simulink model "sim_P_LOS"  (R2017a)
settings: Solver=FixedStepAuto  StartTime=0.0  StopTime=inf  FixedStep=0.01  RelTol=1e-3
values from neighbouring files (symbols this model uses):
  trial_params = sim_params(i)    [exec_sim_main.m]
libraries: simulink x4, emily x1
settings Model: Creator=mitchallain  LastModifiedBy=mitchallain
settings DataIOCC: SaveOutput=off  SaveTime=off

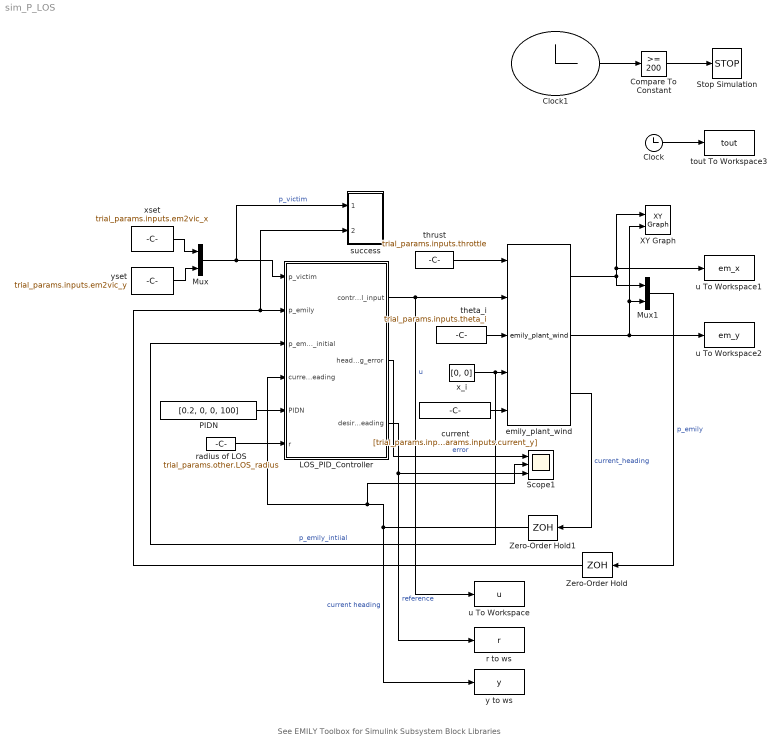
== system sim_P_LOS ==
  note: See EMILY Toolbox for Simulink Subsystem Block Libraries
  Clock : Clock
  Clock1 : Clock
  Compare To Constant : simulink/Logic and Bit Operations/Compare To Constant  relop=>=  const=200  OutDataTypeStr=boolean
  LOS_PID_Controller : Subsystem  AncestorBlock=emily/LOS_PID_Controller
      settings: AttributesFormatString=%<LinkStatus>
  Mux : Mux  Inputs=2
  Mux1 : Mux  Inputs=2
  PIDN : Constant  Value=[0.2, 0, 0, 100]
  Scope1 : Scope  NumInputPorts=3
  Stop Simulation : Stop
  XY Graph : simulink/Sinks/XY Graph  xmin=-50  xmax=50  ymin=-50  ymax=50  st=-1
  Zero-Order Hold : ZeroOrderHold  SampleTime=0.2
  Zero-Order Hold1 : ZeroOrderHold  SampleTime=0.2
  current : Constant  Value=[trial_params.inputs.current_x, trial_params.inputs.current_y]
  emily_plant_wind : emily/emily_plant_wind
      settings: SourceProductName=EMILY Toolbox
  r to ws : ToWorkspace  VariableName=r  SampleTime=0.2
  radius of LOS : Constant  Value=trial_params.other.LOS_radius
  success : Subsystem  AncestorBlock=emily/success
  theta_i : Constant  Value=trial_params.inputs.theta_i
  thrust : Constant  Value=trial_params.inputs.throttle
  tout To Workspace3 : ToWorkspace  VariableName=tout  SampleTime=0.2
  u To Workspace : ToWorkspace  VariableName=u  SampleTime=0.2
  u To Workspace1 : ToWorkspace  VariableName=em_x  SampleTime=0.2
  u To Workspace2 : ToWorkspace  VariableName=em_y  SampleTime=0.2
  x_i : Constant  Value=[0, 0]
  xset : Constant  Value=trial_params.inputs.em2vic_x
  y to ws : ToWorkspace  VariableName=y  SampleTime=0.2
  yset : Constant  Value=trial_params.inputs.em2vic_y
  wires:
  emily_plant_wind/1 -> XY Graph/1, u To Workspace1/1, Mux1/1
  Mux1/1 -> Zero-Order Hold/1  "p_emily"
  thrust/1 -> emily_plant_wind/1
  Mux/1 -> LOS_PID_Controller/1(p_victim), success/1(p_victim)  "p_victim"
  theta_i/1 -> emily_plant_wind/3
  emily_plant_wind/3 -> Zero-Order Hold1/1  "current_heading"
  xset/1 -> Mux/1
  yset/1 -> Mux/2
  emily_plant_wind/2 -> XY Graph/2, Mux1/2, u To Workspace2/1
  LOS_PID_Controller/2(heading_error) -> Scope1/1  "error"
  LOS_PID_Controller/1(control_input) -> emily_plant_wind/2, u To Workspace/1  "u"
  LOS_PID_Controller/3(desired_heading) -> Scope1/3, r to ws/1  "reference"
  x_i/1 -> LOS_PID_Controller/3(p_emily_initial), emily_plant_wind/4  "p_emily_intiial"
  Zero-Order Hold/1 -> LOS_PID_Controller/2(p_emily), success/2(p_emily)
  Zero-Order Hold1/1 -> Scope1/2, LOS_PID_Controller/4(current_heading), y to ws/1  "current heading"
  current/1 -> emily_plant_wind/5
  Clock/1 -> tout To Workspace3/1
  radius of LOS/1 -> LOS_PID_Controller/6(r)
  PIDN/1 -> LOS_PID_Controller/5(PIDN)
  Clock1/1 -> Compare To Constant/1
  Compare To Constant/1 -> Stop Simulation/1

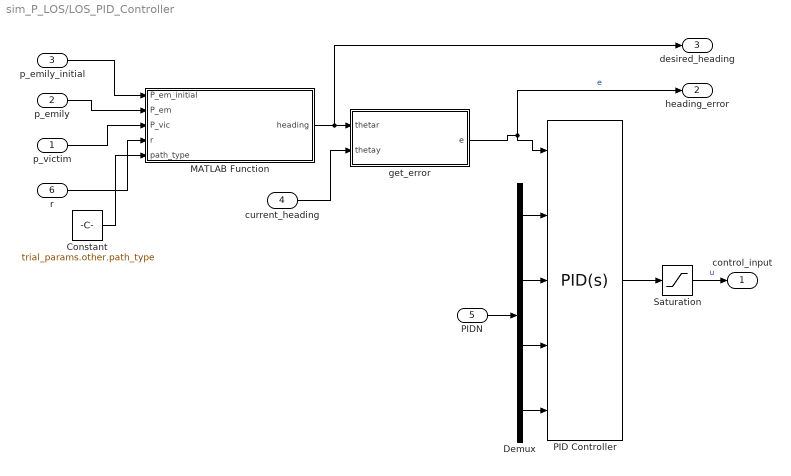
== system sim_P_LOS/LOS_PID_Controller ==
  p_victim : Inport
  p_emily : Inport  Port=2
  p_emily_initial : Inport  Port=3
  current_heading : Inport  Port=4
  PIDN : Inport  Port=5
  r : Inport  Port=6
  Constant : Constant  Value=trial_params.other.path_type  SampleTime=-1
  Demux : Demux
  MATLAB Function : MATLAB Function  TreatAsAtomicUnit=on
  PID Controller : simulink/Continuous/PID Controller  Controller=PID  TimeDomain=Continuous-time  SampleTime=-1  IntegratorMethod=Forward Euler  FilterMethod=Forward Euler  Form=Parallel  UseFilter=on  ControllerParametersSource=external  P=0.01  I=0.0001  D=1  N=100  InitialConditionSource=internal  InitialConditionForIntegrator=0  InitialConditionForFilter=0  ExternalReset=none  LimitOutput=off  UpperSaturationLimit=pi/4  LowerSaturationLimit=-pi/4  LinearizeAsGain=on  AntiWindupMode=clamping  Kb=1  TrackingMode=off  Kt=1  PParamMin=[]  PParamMax=[]  IParamMin=[]  IParamMax=[]  DParamMin=[]  DParamMax=[]  NParamMin=[]  NParamMax=[]  KbParamMin=[]  KbParamMax=[]  KtParamMin=[]  KtParamMax=[]  POutMin=[]  POutMax=[]  IOutMin=[]  IOutMax=[]  DOutMin=[]  DOutMax=[]  NOutMin=[]  NOutMax=[]  KbOutMin=[]  KbOutMax=[]  KtOutMin=[]  KtOutMax=[]  IntegratorOutMin=[]  IntegratorOutMax=[]  FilterOutMin=[]  FilterOutMax=[]  SumOutMin=[]  SumOutMax=[]  SumI1OutMin=[]  SumI1OutMax=[]  SumI2OutMin=[]  SumI2OutMax=[]  SumI3OutMin=[]  SumI3OutMax=[]  SumDOutMin=[]  SumDOutMax=[]  SaturationOutMin=[]  SaturationOutMax=[]  IntegratorContinuousStateAttributes=''  IntegratorStateMustResolveToSignalObject=off  IntegratorRTWStateStorageClass=Auto  FilterContinuousStateAttributes=''  FilterStateMustResolveToSignalObject=off  FilterRTWStateStorageClass=Auto  DifferentiatorICPrevScaledInput=0  DifferentiatorOutMin=[]  DifferentiatorOutMax=[]  InitialConditionSetting=State (most efficient)
  Saturation : Saturate  UpperLimit=pi/4  LowerLimit=-pi/4
  get_error : MATLAB Function  TreatAsAtomicUnit=on
  control_input : Outport
  heading_error : Outport  Port=2
  desired_heading : Outport  Port=3
  wires:
  r/1 -> MATLAB Function/4(r)
  p_emily_initial/1 -> MATLAB Function/1(P_em_initial)
  p_emily/1 -> MATLAB Function/2(P_em)
  p_victim/1 -> MATLAB Function/3(P_vic)
  Demux/4 -> PID Controller/5
  Demux/3 -> PID Controller/4
  Demux/2 -> PID Controller/3
  Demux/1 -> PID Controller/2
  PIDN/1 -> Demux/1
  current_heading/1 -> get_error/2(thetay)
  get_error/1(e) -> PID Controller/1, heading_error/1  "e"
  PID Controller/1 -> Saturation/1
  Saturation/1 -> control_input/1  "u"
  Constant/1 -> MATLAB Function/5(path_type)
  MATLAB Function/1(heading) -> get_error/1(thetar), desired_heading/1

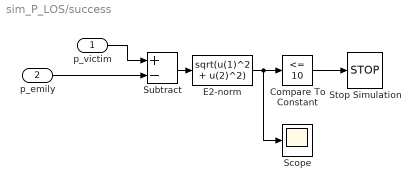
== system sim_P_LOS/success ==
  p_victim : Inport
  p_emily : Inport  Port=2
  Compare To Constant : simulink/Logic and Bit Operations/Compare To Constant  relop=<=  const=10  OutDataTypeStr=boolean
  E2-norm : Fcn  Expr=sqrt(u(1)^2 + u(2)^2)
  Scope : Scope
  Stop Simulation : Stop
  Subtract : Sum  Inputs=+-
  wires:
  Subtract/1 -> E2-norm/1
  E2-norm/1 -> Compare To Constant/1, Scope/1
  p_victim/1 -> Subtract/1
  Compare To Constant/1 -> Stop Simulation/1
  p_emily/1 -> Subtract/2

== matlab function sim_P_LOS/LOS_PID_Controller/get_error ==
  data: thetar input; e output; thetay input
function e  = get_error(thetar, thetay)
%UNTITLED Summary of this function goes here
%   FIX THIS MITCH
e = thetar - thetay;
e = mod((e + pi), 2*pi) - pi;
end

== matlab function sim_P_LOS/LOS_PID_Controller/MATLAB Function ==
  data: P_em_initial input; heading output; P_em input; P_vic input; r input; path_type input
function heading  = straightpathLOS(P_em_initial, P_em, P_vic, r, path_type)
% This function computes the heading angle according to LOS geometric law
%   Assumes straight line path from initial location to victim
%   If two intersections are produced, the intersection with a higher
%   dispacement parameter (s) is chosen (i.e., farther along path)

% Args:
%   P_em_initial (2-vector): initial (x, y) location of EMILY
%   P_em (2-vector): current (x, y) location of EMILY
%   P_vic (2-vector): victim (x, y) location
%   r (float): radius for LOS control

% Returns:
%   heading: heading angle for EMILY in global frame

% Compute vector from initial EMILY to victim in global frame
P_eiv = P_vic - P_em_initial;

% Compute desired path length and angle
d = norm(P_eiv);
path_angle = atan2(P_eiv(2), P_eiv(1));

% Compute vector from current EMILY to victim
P_ev = P_vic - P_em;

% Bearing is used to seed the fminsearch
bearing = atan2(P_ev(2), P_ev(1));

% Parameterized circle about emily
xLOS = @(phi) P_em(1) + r*cos(phi);
yLOS = @(phi) P_em(2) + r*sin(phi);

switch path_type
    case 1
        x = [P_em_initial(1) P_vic(1)/3  P_vic(1)*2/3  P_vic(1)]; %spline intersection pts
        y = [P_em_initial(2) P_vic(2)*2/3  P_vic(2)*2/3  P_vic(2)];
        pp = spline(x,y);
        path = @(s) ppval(pp,s);
        xy = @(param) (path(param(1)) - xLOS(param(2)))^2 + (path(param(1)) - yLOS(param(2)))^2;
        temp = fminsearch(@(param) xy(param), [P_em(1)+20*cos(bearing), bearing]);
        s_i = temp(1);
        phi_i = temp(2);
        P_es = [s_i - P_em(1); path(s_i) - P_em(2)];
        
    case 2
        x = [P_em_initial(1) P_vic(1)/3 P_vic(1)*2/3 P_vic(1)]; %spline intersection pts
        y = [P_em_initial(2) P_em_initial(2)*4/3 P_vic(2)/3  P_vic(2)];
        pp = spline(x,y);
        path = @(s) ppval(pp,s);
        xy = @(param) (path(param(1)) - xLOS(param(2)))^2 + (path(param(1)) - yLOS(param(2)))^2;
        temp = fminsearch(@(param) xy(param), [P_em(1)+20*cos(bearing), bearing]);
        s_i = temp(1);
        phi_i = temp(2);
        P_es = [s_i - P_em(1); path(s_i) - P_em(2)];
        
    case 3
        x = [P_em_initial(1) P_vic(1)/3 P_vic(1)*2/3 P_vic(1)]; %spline intersection pts
        y = [P_em_initial(2) P_vic(2)*2/3 P_em_initial(2)*4/3  P_vic(2)];
        pp = spline(x,y);
        path = @(s) ppval(pp,s);
        xy = @(param) (path(param(1)) - xLOS(param(2)))^2 + (path(param(1)) - yLOS(param(2)))^2;
        temp = fminsearch(@(param) xy(param), [P_em(1)+20*cos(bearing), bearing]);
        s_i = temp(1);
        phi_i = temp(2);
        P_es = [s_i - P_em(1); path(s_i) - P_em(2)];

    otherwise %'straight'
        xpath = @(s) P_em_initial(1) + s*cos(path_angle);
        ypath = @(s) P_em_initial(2) + s*sin(path_angle);
        xy = @(param) (xpath(param(1)) - xLOS(param(2)))^2 + (ypath(param(1)) - yLOS(param(2)))^2;
        temp = fminsearch(@(param) xy(param), [d, bearing]);
        s_i = min(d, max(0, temp(1)));
        phi_i = temp(2);
        P_es = [xpath(s_i) - P_em(1); ypath(s_i) - P_em(2)];
end

heading = atan2(P_es(2), P_es(1));

end
